simulink subsystem "Sensor"  (R2023b)
settings: Solver=VariableStepAuto  StartTime=0.0  StopTime=10.0  RelTol=1e-3
libraries: arduinolib x2
settings Model: Creator=chaya  LastModifiedBy=chaya

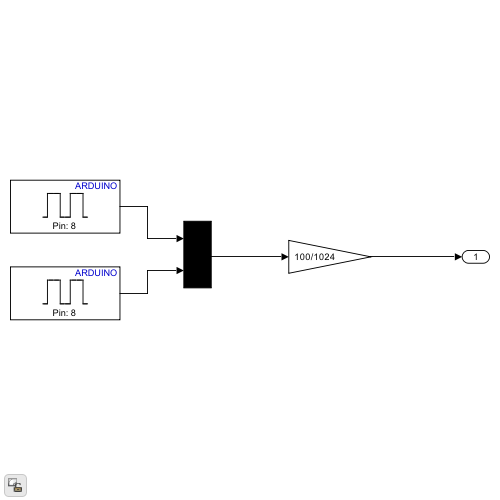
[thumbnail: Simulink's stored preview of the top-level diagram]
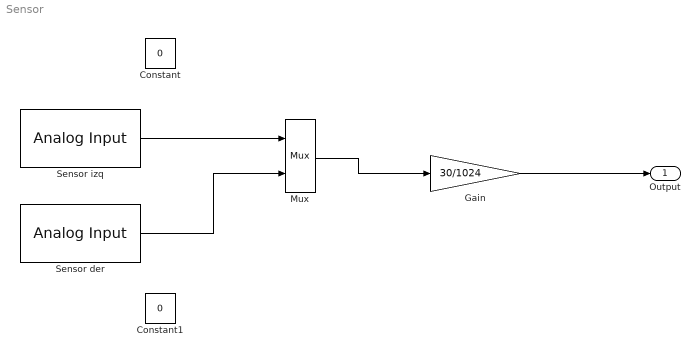
== system Sensor ==
  Constant : Constant  Value=0
  Constant1 : Constant  Value=0
  Gain : Gain  Gain=30/1024
  Mux : Mux  Inputs=2
  Sensor der : arduinolib/Analog Input  pinNumber=0  ReadResultsOnly=off  ConversionTriggerSource=Software  ExternalTriggerType=uint32( 0 )  OutputDataType=uint16  EnableConversionCompleteNotify=off  EnableOuputStatus=off  SampleTime=-1  blockPlatform=arduino
  Sensor izq : arduinolib/Analog Input  pinNumber=1  ReadResultsOnly=off  ConversionTriggerSource=Software  ExternalTriggerType=uint32( 0 )  OutputDataType=uint16  EnableConversionCompleteNotify=off  EnableOuputStatus=off  SampleTime=-1  blockPlatform=arduino
  Output : Outport
  wires:
  Gain/1 -> Output/1
  Mux/1 -> Gain/1
  Sensor izq/1 -> Mux/1
  Sensor der/1 -> Mux/2
